simulink model "q_power_factor_correction"  (R2015a)
settings: Solver=ode45  StartTime=0.0  StopTime=0.7  MaxStep=1/10000  RelTol=1e-3
values from neighbouring files (symbols this model uses):
  k = 0.93    [motor_a2b_param.m]    (also in motor_param.m = 0.796; para.m = 0.5)
  r = 50    [para.m]
  rn = 0.1    [para.m]
libraries: powerlib x17
settings Model: Creator=Windows 10  LastModifiedBy=Windows 10

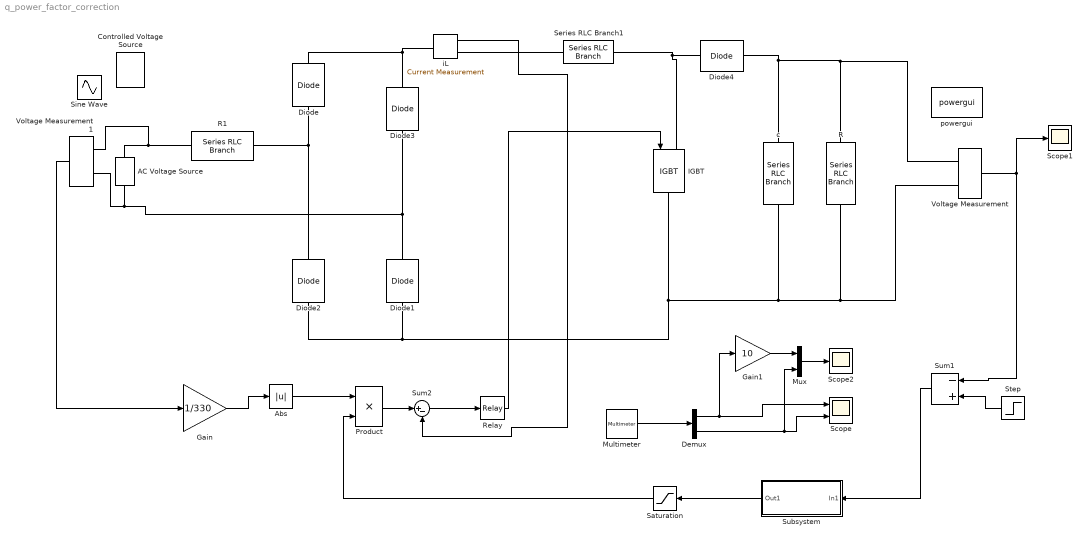
== system q_power_factor_correction ==
  AC Voltage Source : powerlib/Electrical Sources/AC Voltage Source  Amplitude=330  Phase=0  Frequency=50  SampleTime=0  Measurements=Voltage
  Abs : Abs
  Controlled Voltage Source : powerlib/Electrical Sources/Controlled Voltage Source  Initialize=on  Source_Type=AC  Amplitude=0  Phase=0  Frequency=0  Measurements=Voltage
  Demux : Demux  Outputs=2
  Diode{,1..4} (5 alike) : powerlib/Power Electronics/Diode  Ron=0.001  Lon=0  Vf=0.8  IC=0  UseSnubber=off  Rs=500  Cs=250e-9  Measurements=off
  Gain : Gain  Gain=1/330
  Gain1 : Gain  Gain=10
  IGBT : powerlib/Power Electronics/IGBT  Ron=0.001  Lon=0  Vf=1  Tf=1e-6  Tt=2e-6  IC=0  Rs=1e5  Cs=inf  Measurements=off
  Multimeter : powerlib/Measurements/Multimeter  PhasorSimulation=off  OutputType=Complex  sel=[4 2]  L=4  Gain=[1 1]  yselected={'Ib: R1','Usrc: AC Voltage Source'};  PSBOutputType=1  PSBequivalent=0  AxesSetting=[0,0.1,-100,100]  Display=0  SavedBlockNames=-11
  Mux : Mux  Inputs=2
  Product : Product
  R : powerlib/Elements/Series RLC Branch  LConnTagsString=__new0  RConnTagsString=__new0  BranchType=R  Resistance=r  Inductance=1e-3  SetiL0=off  InitialCurrent=0  Capacitance=1e-6  Setx0=off  InitialVoltage=0  Measurements=None
  R1 : powerlib/Elements/Series RLC Branch  LConnTagsString=__new0  RConnTagsString=__new0  BranchType=R  Resistance=rn  Inductance=1e-3  SetiL0=off  InitialCurrent=0  Capacitance=1e-6  Setx0=off  InitialVoltage=0  Measurements=Branch current
  Relay : Relay  OnSwitchValue=0.5  OffSwitchValue=-0.5
  Saturation : Saturate  UpperLimit=60  LowerLimit=-60
  Scope : Scope  NumInputPorts=2
      settings: TimeRange=0.002  YMin=0~40  YMax=40~120
  Scope1 : Scope
  Scope2 : Scope
      settings: SaveName=ScopeData2
  Series RLC Branch1 : powerlib/Elements/Series RLC Branch  LConnTagsString=__new0  RConnTagsString=__new0  BranchType=L  Resistance=5  Inductance=5/1000  SetiL0=off  InitialCurrent=0  Capacitance=1e-6  Setx0=off  InitialVoltage=0  Measurements=Branch voltage
  Sine Wave : Sin  Amplitude=330  Frequency=50  SampleTime=0
  Step : Step  Time=0.3  Before=400  After=500  SampleTime=0
  Subsystem : Subsystem
  Sum1 : Sum  Inputs=-+
  Sum2 : Sum  Inputs=|+-
  Voltage Measurement : powerlib/Measurements/Voltage Measurement  PhasorSimulation=off  OutputType=Complex  PSBequivalent=0
  Voltage Measurement1 : powerlib/Measurements/Voltage Measurement  PhasorSimulation=off  OutputType=Complex  PSBequivalent=0
  c : powerlib/Elements/Series RLC Branch  LConnTagsString=__new0  RConnTagsString=__new0  BranchType=C  Resistance=5  Inductance=1e-3  SetiL0=off  InitialCurrent=0  Capacitance=5/1000  Setx0=on  InitialVoltage=uc0  Measurements=None
  iL : powerlib/Measurements/Current Measurement  PhasorSimulation=off  OutputType=Complex  PSBequivalent=0
  powergui : powerlib/powergui  Priority=1  SimulationMode=Continuous  SolverType=Tustin/Backward Euler (TBE)  SampleTime=50e-6  frequency=60  SPID=off  DisableSnubberDevices=off  DisableRonSwitches=off  DisableVfSwitches=off  SwTol=0  DisplayEquations=off  Interpol=off  methode=off  Ts=100  FunctionMessages=off  echomessages=off  HookPort=off  EnableUseOfTLC=off  x0status=blocks  frequencyindice=0  Pbase=100e6  ErrMax=1e-4  Iterations=50  UnitsV=kV  UnitsW=MW  buscounter=0  RestoreLinks=warning  ResistiveCurrentMeasurement=off  Frange=[0:2:500]  Ylog=off  Xlog=on  ShowGrid=off  save=off  variable=ZData  structure=0  ZoomFFT=off  StartTime=0.0  cycles=1  DisplayStyle=1  fundamental=60  FreqAxis=off  MaxFrequency=1000  frequencyindicesteady=1  RmsSteady=1  display=off
  wires:
  Gain/1 -> Abs/1
  Abs/1 -> Product/1
  Product/1 -> Sum2/1
  Sum2/1 -> Relay/1
  Relay/1 -> IGBT/1
  Sum1/1 -> Subsystem/1(In1)
  Step/1 -> Sum1/2
  Voltage Measurement/1 -> Sum1/1, Scope1/1
  Subsystem/1(Out1) -> Saturation/1
  Saturation/1 -> Product/2
  Multimeter/1 -> Demux/1
  Demux/2 -> Mux/2, Scope/2
  Demux/1 -> Gain1/1, Scope/1
  iL/1 -> Sum2/2
  Voltage Measurement1/1 -> Gain/1
  Mux/1 -> Scope2/1
  Gain1/1 -> Mux/1
  connections:
  Diode2/RConn1 -- R1/RConn1 -- Diode/LConn1
  Diode1/RConn1 -- AC Voltage Source/LConn1 -- Voltage Measurement1/LConn2 -- Diode3/LConn1
  Diode2/LConn1 -- IGBT/RConn1 -- Voltage Measurement/LConn2 -- R/RConn1 -- c/RConn1 -- Diode1/LConn1
  Diode/RConn1 -- Diode3/RConn1 -- iL/LConn1
  AC Voltage Source/RConn1 -- Voltage Measurement1/LConn1 -- R1/LConn1
  iL/RConn1 -- Series RLC Branch1/LConn1
  Series RLC Branch1/RConn1 -- IGBT/LConn1 -- Diode4/LConn1
  c/LConn1 -- Voltage Measurement/LConn1 -- R/LConn1 -- Diode4/RConn1

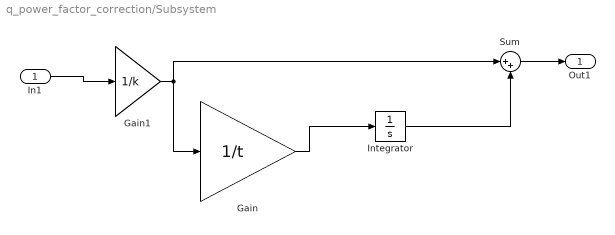
== system q_power_factor_correction/Subsystem ==
  In1 : Inport
  Gain : Gain  Gain=1/t
  Gain1 : Gain  Gain=1/k
  Integrator : Integrator
  Sum : Sum  Inputs=|++
  Out1 : Outport
  wires:
  In1/1 -> Gain1/1
  Gain/1 -> Integrator/1
  Integrator/1 -> Sum/2
  Gain1/1 -> Sum/1, Gain/1
  Sum/1 -> Out1/1
